simulink model "MF2"  (R2017b)
settings: Solver=VariableStepAuto  StartTime=0.0  StopTime=50  RelTol=1e-3
settings Model: Creator=Cx001la  LastModifiedBy=Cx001la

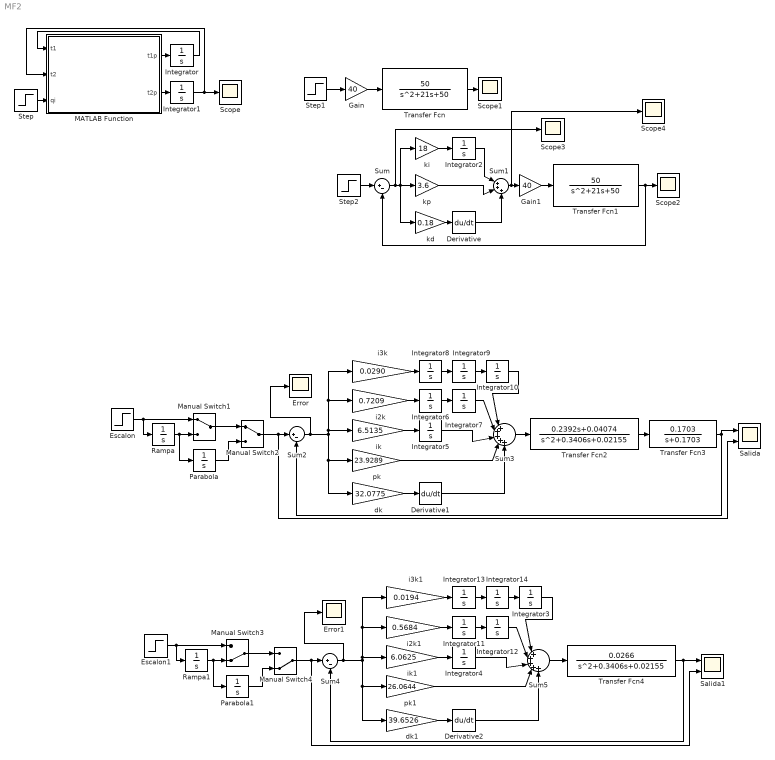
== system MF2 ==
  Derivative : Derivative
  Derivative1 : Derivative
  Derivative2 : Derivative
  Error : Scope
  Error1 : Scope
  Escalon : Step  Time=0  SampleTime=0
  Escalon1 : Step  Time=0  SampleTime=0
  Gain : Gain  Gain=40
  Gain1 : Gain  Gain=40
  Integrator{,1..14} (15 alike) : Integrator
  MATLAB Function : MATLAB Function  TreatAsAtomicUnit=on
  Manual Switch1 : ManualSwitch
  Manual Switch2 : ManualSwitch
  Manual Switch3 : ManualSwitch  CurrentSetting=0
  Manual Switch4 : ManualSwitch  CurrentSetting=0
  Parabola : Integrator
  Parabola1 : Integrator
  Rampa : Integrator
  Rampa1 : Integrator
  Salida : Scope  NumInputPorts=2
  Salida1 : Scope  NumInputPorts=2
  Scope{,1..4} (5 alike) : Scope
  Step : Step  SampleTime=0
  Step1 : Step  Time=0  SampleTime=0
  Step2 : Step  Time=0  After=400  SampleTime=0
  Sum : Sum  Inputs=|+-
  Sum1 : Sum  Inputs=|+++
  Sum2 : Sum  Inputs=|+-
  Sum3 : Sum  Inputs=|+++++
  Sum4 : Sum  Inputs=|+-
  Sum5 : Sum  Inputs=|+++++
  Transfer Fcn : TransferFcn  Numerator=[50]  Denominator=[1 21 50]
  Transfer Fcn1 : TransferFcn  Numerator=[50]  Denominator=[1 21 50]
  Transfer Fcn2 : TransferFcn  Numerator=[0.2392 0.04074]  Denominator=[1 0.3406 0.02155]
  Transfer Fcn3 : TransferFcn  Numerator=[0.1703]  Denominator=[1 0.1703]
  Transfer Fcn4 : TransferFcn  Numerator=[0.0266]  Denominator=[1 0.3406 0.02155]
  dk : Gain  Gain=32.0775
  dk1 : Gain  Gain=39.6526
  i2k : Gain  Gain=0.7209
  i2k1 : Gain  Gain=0.5684
  i3k : Gain  Gain=0.0290
  i3k1 : Gain  Gain=0.0194
  ik : Gain  Gain=6.5135
  ik1 : Gain  Gain=6.0625
  kd : Gain  Gain=0.18
  ki : Gain  Gain=18
  kp : Gain  Gain=3.6
  pk : Gain  Gain=23.9289
  pk1 : Gain  Gain=26.0644
  wires:
  MATLAB Function/2(t2p) -> Integrator1/1
  MATLAB Function/1(t1p) -> Integrator/1
  Integrator/1 -> MATLAB Function/1(t1)
  Integrator1/1 -> Scope/1, MATLAB Function/2(t2)
  Step/1 -> MATLAB Function/3(qi)
  Transfer Fcn/1 -> Scope1/1
  Gain/1 -> Transfer Fcn/1
  Step1/1 -> Gain/1
  Gain1/1 -> Transfer Fcn1/1
  Transfer Fcn1/1 -> Scope2/1, Sum/2
  Step2/1 -> Sum/1
  Sum/1 -> Scope3/1, kd/1, ki/1, kp/1
  ki/1 -> Integrator2/1
  kd/1 -> Derivative/1
  kp/1 -> Sum1/2
  Sum1/1 -> Scope4/1, Gain1/1
  Derivative/1 -> Sum1/3
  Integrator2/1 -> Sum1/1
  Sum2/1 -> Error/1, i3k/1, i2k/1, ik/1, pk/1, dk/1
  dk/1 -> Derivative1/1
  ik/1 -> Integrator5/1
  Integrator6/1 -> Integrator7/1
  i2k/1 -> Integrator6/1
  Integrator8/1 -> Integrator9/1
  i3k/1 -> Integrator8/1
  Integrator9/1 -> Integrator10/1
  Integrator10/1 -> Sum3/1
  Integrator7/1 -> Sum3/2
  Integrator5/1 -> Sum3/3
  pk/1 -> Sum3/4
  Derivative1/1 -> Sum3/5
  Transfer Fcn3/1 -> Sum2/2, Salida/1
  Sum3/1 -> Transfer Fcn2/1
  Transfer Fcn2/1 -> Transfer Fcn3/1
  Escalon/1 -> Rampa/1, Manual Switch1/1
  Rampa/1 -> Parabola/1, Manual Switch1/2
  Manual Switch2/1 -> Salida/2, Sum2/1
  Manual Switch1/1 -> Manual Switch2/1
  Parabola/1 -> Manual Switch2/2
  Manual Switch3/1 -> Manual Switch4/1
  Manual Switch4/1 -> Salida1/2, Sum4/1
  i2k1/1 -> Integrator11/1
  Sum4/1 -> Error1/1, i3k1/1, i2k1/1, ik1/1, pk1/1, dk1/1
  Derivative2/1 -> Sum5/5
  Integrator13/1 -> Integrator14/1
  Integrator3/1 -> Sum5/1
  Integrator4/1 -> Sum5/3
  i3k1/1 -> Integrator13/1
  Integrator12/1 -> Sum5/2
  ik1/1 -> Integrator4/1
  Integrator14/1 -> Integrator3/1
  dk1/1 -> Derivative2/1
  Integrator11/1 -> Integrator12/1
  Escalon1/1 -> Rampa1/1, Manual Switch3/1
  Transfer Fcn4/1 -> Sum4/2, Salida1/1
  pk1/1 -> Sum5/4
  Parabola1/1 -> Manual Switch4/2
  Rampa1/1 -> Parabola1/1, Manual Switch3/2
  Sum5/1 -> Transfer Fcn4/1

== matlab function MF2/MATLAB Function ==
  data: t1 input; t1p output; t2 input; qi input; t2p output
function [t1p,t2p] = fcn(t1,t2,qi)
c1=0.005; c2=0.002;  r1=50; r2=100; ta=293;

q1=(t1-ta)/r2;
q2=(t1-t2)/r1;
q3=(t2-ta)/r2;
t1p=(qi-q1-q2)/c1;
t2p=(q2-q3)/c2;
